simulink model "AUAV_V3_TestSensors_"  (R2015a)
settings: Solver=FixedStepDiscrete  StartTime=0.0  StopTime=10.0  FixedStep=T  RelTol=1e-3
PreLoadFcn:
  | %T = 0.0025;
  | MavlinkBus;
  | mcuInit;
  | % Baro Altitude Computation
  | % =========================
  | basePressure = 98192.64;
  | baseTemp = 288.215;
  | lapseRate = -0.00198122;
  | baseHeight = 0;
values from neighbouring files (symbols this model uses):
  apSampleTime = 0.01    [mcuInit.m]
  latlong_WP = 1    [mcuInit.m]
  mavlink_attitude_t = Simulink.Bus    [MavlinkBusMarcello.m]
  mavlink_gps_raw_int_t = Simulink.Bus    [MavlinkBus.m]    (also in MavlinkBusMarcello.m)
  mavlink_raw_imu_t = Simulink.Bus    [MavlinkBus.m]    (also in MavlinkBusMarcello.m)
  mavlink_scaled_pressure_t = Simulink.Bus    [MavlinkBus.m]    (also in MavlinkBusMarcello.m)
  mavlink_servo_output_raw_t = Simulink.Bus    [MavlinkBusMarcello.m]
  mavlink_sys_status_t = Simulink.Bus    [MavlinkBus.m]    (also in MavlinkBusMarcello.m)
  T = 0.01    [mcuInit.m]
  Xpoints = [0 0]    [mcuInit.m]
  Ypoints = [0 0]    [mcuInit.m]
  Zpoints = [0 0]    [mcuInit.m]
undefined symbols (not defined in the file or in its folder): A0, A14, A15, A2, A3, A4, A5, A6, accBiasRateLimit, B0, bankCommandLimit, barAdjust, baroCutoff, baroCutTemp, cubeAccelGain16405, cubeGyroGain16405, cubeMagGain16405, D0, D11, D7, D8, daLimit, data, daTrimMax, daTrimMin, deLimit, deTrimMax, deTrimMin, drLimit, drTrimMax, drTrimMin, dtLimit, dtTrimMax, dtTrimMin, F2, F3, G0, G13, G15, gaind, GS_location, gyroBiasRateLimit, IC1max, IPStar, ISA_g, Max, maxAcc, MaxDwnPthStar, maxDynPressure, maxEta, mlParamInterface, ms, OC1max, P112, P125, P127, P16, P20, P21, P30 ... (+26)
undefined symbols (not defined in the file): baroOffset, baroScale, barTGain1, barTGain2, barTMean1, barTMean2, bda, bde, bdr, bdt, bICda, bICde, bICdr, bICdt, derivativesConstant, lowRateSensorCutoff, mainSensorCutoff, mda, mde, mdr, mdt, mICda, mICde, mICdr, mICdt, pitotOffset, pitotScale, pitTGain1, pitTGain2, pitTMean1, pitTMean2, powerOffset, powerScale, pressureSensorCutoff, tempOffset, tempScale, vzCutoff, xCutoff, yCutoff
libraries: MCHP_Blockset x150, simulink x84, SLUGS_Library x31, aerolibconvert2 x6, aerolibutil x4, aerolibtransform2 x3, dspmtrx3 x2, aerolibobsolete x2
(part 11 of 20)

== system AUAV_V3_TestSensors_/Barometer_Driver/Baro Altimeter/Zero Out Height ==
  Base Height : Inport
  Computed Height : Inport  Port=2
  Enable : EnablePort
  Integer Delay : Delay  DelayLength=1  InitialCondition=0  InputProcessing=Inherited  SampleTime=.01
  Sum : Sum  Inputs=|+-  OutDataTypeStr=single
  Height Offset : Outport
  wires:
  Base Height/1 -> Sum/1
  Integer Delay/1 -> Sum/2
  Sum/1 -> Height Offset/1
  Computed Height/1 -> Integer Delay/1

== system AUAV_V3_TestSensors_/Barometer_Driver/I2C Initialisation Read EEPROM Calibration data Once (Blocking Function)/Pack10 ==
  Hi : Inport
  Low : Inport  Port=2
  Bitwise Operator : simulink/Logic and Bit Operations/Bitwise Operator  logicop=OR  UseBitMask=off  NumInputPorts=2  BitMask=bin2dec('11011001')  BitMaskRealWorld=Stored Integer
  Data Type Conversion1 : DataTypeConversion  OutDataTypeStr=uint16  ConvertRealWorld=Stored Integer (SI)
  Data Type Conversion2 : DataTypeConversion  OutDataTypeStr=uint16  ConvertRealWorld=Stored Integer (SI)
  Data Type Conversion3 : DataTypeConversion  OutDataTypeStr=uint16  ConvertRealWorld=Stored Integer (SI)
  Gain : Gain  Gain=2^8  OutDataTypeStr=Inherit: Same as input
  Out1 : Outport
  wires:
  Data Type Conversion3/1 -> Bitwise Operator/2
  Low/1 -> Data Type Conversion3/1
  Data Type Conversion1/1 -> Gain/1
  Bitwise Operator/1 -> Data Type Conversion2/1
  Hi/1 -> Data Type Conversion1/1
  Gain/1 -> Bitwise Operator/1
  Data Type Conversion2/1 -> Out1/1

== system AUAV_V3_TestSensors_/Barometer_Driver/I2C Initialisation Read EEPROM Calibration data Once (Blocking Function)/Pack11 ==
  Hi : Inport
  Low : Inport  Port=2
  Bitwise Operator : simulink/Logic and Bit Operations/Bitwise Operator  logicop=OR  UseBitMask=off  NumInputPorts=2  BitMask=bin2dec('11011001')  BitMaskRealWorld=Stored Integer
  Data Type Conversion1 : DataTypeConversion  OutDataTypeStr=uint16  ConvertRealWorld=Stored Integer (SI)
  Data Type Conversion2 : DataTypeConversion  OutDataTypeStr=uint16  ConvertRealWorld=Stored Integer (SI)
  Data Type Conversion3 : DataTypeConversion  OutDataTypeStr=uint16  ConvertRealWorld=Stored Integer (SI)
  Gain : Gain  Gain=2^8  OutDataTypeStr=Inherit: Same as input
  Out1 : Outport
  wires:
  Data Type Conversion3/1 -> Bitwise Operator/2
  Low/1 -> Data Type Conversion3/1
  Data Type Conversion1/1 -> Gain/1
  Bitwise Operator/1 -> Data Type Conversion2/1
  Hi/1 -> Data Type Conversion1/1
  Gain/1 -> Bitwise Operator/1
  Data Type Conversion2/1 -> Out1/1

== system AUAV_V3_TestSensors_/Barometer_Driver/I2C Initialisation Read EEPROM Calibration data Once (Blocking Function)/Pack12 ==
  Hi : Inport
  Low : Inport  Port=2
  Bitwise Operator : simulink/Logic and Bit Operations/Bitwise Operator  logicop=OR  UseBitMask=off  NumInputPorts=2  BitMask=bin2dec('11011001')  BitMaskRealWorld=Stored Integer
  Data Type Conversion1 : DataTypeConversion  OutDataTypeStr=uint16  ConvertRealWorld=Stored Integer (SI)
  Data Type Conversion2 : DataTypeConversion  OutDataTypeStr=uint16  ConvertRealWorld=Stored Integer (SI)
  Data Type Conversion3 : DataTypeConversion  OutDataTypeStr=uint16  ConvertRealWorld=Stored Integer (SI)
  Gain : Gain  Gain=2^8  OutDataTypeStr=Inherit: Same as input
  Out1 : Outport
  wires:
  Data Type Conversion2/1 -> Out1/1
  Gain/1 -> Bitwise Operator/1
  Hi/1 -> Data Type Conversion1/1
  Bitwise Operator/1 -> Data Type Conversion2/1
  Data Type Conversion1/1 -> Gain/1
  Low/1 -> Data Type Conversion3/1
  Data Type Conversion3/1 -> Bitwise Operator/2

== system AUAV_V3_TestSensors_/Barometer_Driver/I2C Initialisation Read EEPROM Calibration data Once (Blocking Function)/Pack2 ==
  Hi : Inport
  Low : Inport  Port=2
  Bitwise Operator : simulink/Logic and Bit Operations/Bitwise Operator  logicop=OR  UseBitMask=off  NumInputPorts=2  BitMask=bin2dec('11011001')  BitMaskRealWorld=Stored Integer
  Data Type Conversion1 : DataTypeConversion  OutDataTypeStr=uint16  ConvertRealWorld=Stored Integer (SI)
  Data Type Conversion2 : DataTypeConversion  OutDataTypeStr=uint16  ConvertRealWorld=Stored Integer (SI)
  Data Type Conversion3 : DataTypeConversion  OutDataTypeStr=uint16  ConvertRealWorld=Stored Integer (SI)
  Gain : Gain  Gain=2^8  OutDataTypeStr=Inherit: Same as input
  Out1 : Outport
  wires:
  Data Type Conversion2/1 -> Out1/1
  Gain/1 -> Bitwise Operator/1
  Hi/1 -> Data Type Conversion1/1
  Bitwise Operator/1 -> Data Type Conversion2/1
  Data Type Conversion1/1 -> Gain/1
  Low/1 -> Data Type Conversion3/1
  Data Type Conversion3/1 -> Bitwise Operator/2

== system AUAV_V3_TestSensors_/Barometer_Driver/I2C Initialisation Read EEPROM Calibration data Once (Blocking Function)/Pack3 ==
  Hi : Inport
  Low : Inport  Port=2
  Bitwise Operator : simulink/Logic and Bit Operations/Bitwise Operator  logicop=OR  UseBitMask=off  NumInputPorts=2  BitMask=bin2dec('11011001')  BitMaskRealWorld=Stored Integer
  Data Type Conversion1 : DataTypeConversion  OutDataTypeStr=uint16  ConvertRealWorld=Stored Integer (SI)
  Data Type Conversion2 : DataTypeConversion  OutDataTypeStr=uint16  ConvertRealWorld=Stored Integer (SI)
  Data Type Conversion3 : DataTypeConversion  OutDataTypeStr=uint16  ConvertRealWorld=Stored Integer (SI)
  Gain : Gain  Gain=2^8  OutDataTypeStr=Inherit: Same as input
  Out1 : Outport
  wires:
  Data Type Conversion3/1 -> Bitwise Operator/2
  Low/1 -> Data Type Conversion3/1
  Data Type Conversion1/1 -> Gain/1
  Bitwise Operator/1 -> Data Type Conversion2/1
  Hi/1 -> Data Type Conversion1/1
  Gain/1 -> Bitwise Operator/1
  Data Type Conversion2/1 -> Out1/1

== system AUAV_V3_TestSensors_/Barometer_Driver/I2C Initialisation Read EEPROM Calibration data Once (Blocking Function)/Pack4 ==
  Hi : Inport
  Low : Inport  Port=2
  Bitwise Operator : simulink/Logic and Bit Operations/Bitwise Operator  logicop=OR  UseBitMask=off  NumInputPorts=2  BitMask=bin2dec('11011001')  BitMaskRealWorld=Stored Integer
  Data Type Conversion1 : DataTypeConversion  OutDataTypeStr=uint16  ConvertRealWorld=Stored Integer (SI)
  Data Type Conversion2 : DataTypeConversion  OutDataTypeStr=uint16  ConvertRealWorld=Stored Integer (SI)
  Data Type Conversion3 : DataTypeConversion  OutDataTypeStr=uint16  ConvertRealWorld=Stored Integer (SI)
  Gain : Gain  Gain=2^8  OutDataTypeStr=Inherit: Same as input
  Out1 : Outport
  wires:
  Data Type Conversion3/1 -> Bitwise Operator/2
  Low/1 -> Data Type Conversion3/1
  Data Type Conversion1/1 -> Gain/1
  Bitwise Operator/1 -> Data Type Conversion2/1
  Hi/1 -> Data Type Conversion1/1
  Gain/1 -> Bitwise Operator/1
  Data Type Conversion2/1 -> Out1/1

== system AUAV_V3_TestSensors_/Barometer_Driver/I2C Initialisation Read EEPROM Calibration data Once (Blocking Function)/Pack5 ==
  Hi : Inport
  Low : Inport  Port=2
  Bitwise Operator : simulink/Logic and Bit Operations/Bitwise Operator  logicop=OR  UseBitMask=off  NumInputPorts=2  BitMask=bin2dec('11011001')  BitMaskRealWorld=Stored Integer
  Data Type Conversion1 : DataTypeConversion  OutDataTypeStr=uint16  ConvertRealWorld=Stored Integer (SI)
  Data Type Conversion2 : DataTypeConversion  OutDataTypeStr=uint16  ConvertRealWorld=Stored Integer (SI)
  Data Type Conversion3 : DataTypeConversion  OutDataTypeStr=uint16  ConvertRealWorld=Stored Integer (SI)
  Gain : Gain  Gain=2^8  OutDataTypeStr=Inherit: Same as input
  Out1 : Outport
  wires:
  Data Type Conversion2/1 -> Out1/1
  Gain/1 -> Bitwise Operator/1
  Hi/1 -> Data Type Conversion1/1
  Bitwise Operator/1 -> Data Type Conversion2/1
  Data Type Conversion1/1 -> Gain/1
  Low/1 -> Data Type Conversion3/1
  Data Type Conversion3/1 -> Bitwise Operator/2

== system AUAV_V3_TestSensors_/Barometer_Driver/I2C Initialisation Read EEPROM Calibration data Once (Blocking Function)/Pack6 ==
  Hi : Inport
  Low : Inport  Port=2
  Bitwise Operator : simulink/Logic and Bit Operations/Bitwise Operator  logicop=OR  UseBitMask=off  NumInputPorts=2  BitMask=bin2dec('11011001')  BitMaskRealWorld=Stored Integer
  Data Type Conversion1 : DataTypeConversion  OutDataTypeStr=uint16  ConvertRealWorld=Stored Integer (SI)
  Data Type Conversion2 : DataTypeConversion  OutDataTypeStr=uint16  ConvertRealWorld=Stored Integer (SI)
  Data Type Conversion3 : DataTypeConversion  OutDataTypeStr=uint16  ConvertRealWorld=Stored Integer (SI)
  Gain : Gain  Gain=2^8  OutDataTypeStr=Inherit: Same as input
  Out1 : Outport
  wires:
  Data Type Conversion3/1 -> Bitwise Operator/2
  Low/1 -> Data Type Conversion3/1
  Data Type Conversion1/1 -> Gain/1
  Bitwise Operator/1 -> Data Type Conversion2/1
  Hi/1 -> Data Type Conversion1/1
  Gain/1 -> Bitwise Operator/1
  Data Type Conversion2/1 -> Out1/1

== system AUAV_V3_TestSensors_/Barometer_Driver/I2C Initialisation Read EEPROM Calibration data Once (Blocking Function)/Pack7 ==
  Hi : Inport
  Low : Inport  Port=2
  Bitwise Operator : simulink/Logic and Bit Operations/Bitwise Operator  logicop=OR  UseBitMask=off  NumInputPorts=2  BitMask=bin2dec('11011001')  BitMaskRealWorld=Stored Integer
  Data Type Conversion1 : DataTypeConversion  OutDataTypeStr=uint16  ConvertRealWorld=Stored Integer (SI)
  Data Type Conversion2 : DataTypeConversion  OutDataTypeStr=uint16  ConvertRealWorld=Stored Integer (SI)
  Data Type Conversion3 : DataTypeConversion  OutDataTypeStr=uint16  ConvertRealWorld=Stored Integer (SI)
  Gain : Gain  Gain=2^8  OutDataTypeStr=Inherit: Same as input
  Out1 : Outport
  wires:
  Data Type Conversion2/1 -> Out1/1
  Gain/1 -> Bitwise Operator/1
  Hi/1 -> Data Type Conversion1/1
  Bitwise Operator/1 -> Data Type Conversion2/1
  Data Type Conversion1/1 -> Gain/1
  Low/1 -> Data Type Conversion3/1
  Data Type Conversion3/1 -> Bitwise Operator/2

== system AUAV_V3_TestSensors_/Barometer_Driver/I2C Initialisation Read EEPROM Calibration data Once (Blocking Function)/Pack8 ==
  Hi : Inport
  Low : Inport  Port=2
  Bitwise Operator : simulink/Logic and Bit Operations/Bitwise Operator  logicop=OR  UseBitMask=off  NumInputPorts=2  BitMask=bin2dec('11011001')  BitMaskRealWorld=Stored Integer
  Data Type Conversion1 : DataTypeConversion  OutDataTypeStr=uint16  ConvertRealWorld=Stored Integer (SI)
  Data Type Conversion2 : DataTypeConversion  OutDataTypeStr=uint16  ConvertRealWorld=Stored Integer (SI)
  Data Type Conversion3 : DataTypeConversion  OutDataTypeStr=uint16  ConvertRealWorld=Stored Integer (SI)
  Gain : Gain  Gain=2^8  OutDataTypeStr=Inherit: Same as input
  Out1 : Outport
  wires:
  Data Type Conversion2/1 -> Out1/1
  Gain/1 -> Bitwise Operator/1
  Hi/1 -> Data Type Conversion1/1
  Bitwise Operator/1 -> Data Type Conversion2/1
  Data Type Conversion1/1 -> Gain/1
  Low/1 -> Data Type Conversion3/1
  Data Type Conversion3/1 -> Bitwise Operator/2

== system AUAV_V3_TestSensors_/Barometer_Driver/I2C Initialisation Read EEPROM Calibration data Once (Blocking Function)/Pack9 ==
  Hi : Inport
  Low : Inport  Port=2
  Bitwise Operator : simulink/Logic and Bit Operations/Bitwise Operator  logicop=OR  UseBitMask=off  NumInputPorts=2  BitMask=bin2dec('11011001')  BitMaskRealWorld=Stored Integer
  Data Type Conversion1 : DataTypeConversion  OutDataTypeStr=uint16  ConvertRealWorld=Stored Integer (SI)
  Data Type Conversion2 : DataTypeConversion  OutDataTypeStr=uint16  ConvertRealWorld=Stored Integer (SI)
  Data Type Conversion3 : DataTypeConversion  OutDataTypeStr=uint16  ConvertRealWorld=Stored Integer (SI)
  Gain : Gain  Gain=2^8  OutDataTypeStr=Inherit: Same as input
  Out1 : Outport
  wires:
  Data Type Conversion3/1 -> Bitwise Operator/2
  Low/1 -> Data Type Conversion3/1
  Data Type Conversion1/1 -> Gain/1
  Bitwise Operator/1 -> Data Type Conversion2/1
  Hi/1 -> Data Type Conversion1/1
  Gain/1 -> Bitwise Operator/1
  Data Type Conversion2/1 -> Out1/1

== system AUAV_V3_TestSensors_/Control Surface Input/PilotConsole/Convert to Microseconds  ==
  IC : Inport
  Convert to Microseconds : Gain  Gain=0.2
  Data Type Conversion : DataTypeConversion  OutDataTypeStr=uint16
  uS : Outport
  wires:
  Convert to Microseconds/1 -> Data Type Conversion/1
  IC/1 -> Convert to Microseconds/1
  Data Type Conversion/1 -> uS/1

== system AUAV_V3_TestSensors_/Inner Loop// Navigation/Compute psi_dot_m/Protect NaNs ==
  In1 : Inport
  Integer Delay3 : Delay  DelayLength=1  InputProcessing=Inherited  SampleTime=T
  Relational Operator2 : RelationalOperator  Operator===  OutDataTypeStr=uint(8)
  Switch3 : Switch  Criteria=u2 > Threshold  Threshold=0.3  SampleTime=.01
  Out1 : Outport
  wires:
  Integer Delay3/1 -> Switch3/3
  Switch3/1 -> Out1/1, Integer Delay3/1
  In1/1 -> Relational Operator2/2, Relational Operator2/1, Switch3/1
  Relational Operator2/1 -> Switch3/2

== system AUAV_V3_TestSensors_/Inner Loop// Navigation/Compute psi_dot_m/dsPIC_cos ==
  u : Inport
  Environment Controller1 : simulink/Signal Routing/Environment Controller
  Trigonometric Function : Trigonometry  Operator=cos
  myCos() aLib.c [updated 5.1.16] : MCHP_Blockset/User Functions/C Function Call  ParseFilesChkbx=off  ListFunctions1=Custom Function  Function1=float myCos(float x)  AddHeaderDeclaration=off  Function1Type=when block is updated (default)  Fct1BlockIn=x  FctReturnBlockOut=on  DataCollected=0  ORDERING=None  SampleTime=-1  MCHP_MASTERLINK=|  PinDigitalInput=[]  PinDigitalOutput=[]  PinAnalogInput=[]
      | AUAV_V3_TestSensors_/Microchip Master
      | AUAV V3 Board
      | Busy Flag on D2 (RA6)
  cos(u) : Outport
  wires:
  u/1 -> Trigonometric Function/1, myCos() aLib.c [updated 5.1.16]/1
  Environment Controller1/1 -> cos(u)/1
  Trigonometric Function/1 -> Environment Controller1/1
  myCos() aLib.c [updated 5.1.16]/1 -> Environment Controller1/2

== system AUAV_V3_TestSensors_/Inner Loop// Navigation/Compute psi_dot_m/dsPIC_sin ==
  note: mySin()
      | alib.c
      | [updated 5.1.16]
  x : Inport
  C Function Call1 : MCHP_Blockset/User Functions/C Function Call  ParseFilesChkbx=off  ListFunctions1=Custom Function  Function1=float mySin(float x)  AddHeaderDeclaration=off  Function1Type=when block is updated (default)  Fct1BlockIn=x  FctReturnBlockOut=on  DataCollected=0  ORDERING=None  SampleTime=-1  MCHP_MASTERLINK=|  PinDigitalInput=[]  PinDigitalOutput=[]  PinAnalogInput=[]
      | AUAV_V3_TestSensors_/Microchip Master
      | AUAV V3 Board
      | Busy Flag on D2 (RA6)
  Environment Controller : simulink/Signal Routing/Environment Controller
  Trigonometric Function : Trigonometry
  sin(x) : Outport
  wires:
  x/1 -> Trigonometric Function/1, C Function Call1/1
  Trigonometric Function/1 -> Environment Controller/1
  Environment Controller/1 -> sin(x)/1
  C Function Call1/1 -> Environment Controller/2

== system AUAV_V3_TestSensors_/Inner Loop// Navigation/L1 Output Feedback Controller With Projection Operator/Control Law ==
  a : Inport
  u : Inport  Port=2
  Compute Coef : Subsystem
  Detect Change : Subsystem
  Divide : Product  SampleTime=apSampleTime
  Divide1 : Product  SampleTime=apSampleTime
  IC : InitialCondition
  Integer Delay : Delay  DelayLength=1  InputProcessing=Inherited  SampleTime=apSampleTime
  Integer Delay1 : Delay  DelayLength=1  InputProcessing=Inherited  SampleTime=apSampleTime
  Subtract : Sum  SampleTime=apSampleTime
  y : Outport
  wires:
  a/1 -> Compute Coef/1(a), Detect Change/1(Data)
  Compute Coef/1(b) -> Divide/1
  Compute Coef/2(c) -> Divide1/1
  Detect Change/1(change?) -> IC/1
  Integer Delay/1 -> Divide/2
  Divide/1 -> Subtract/1
  Divide1/1 -> Subtract/2
  Subtract/1 -> y/1, Integer Delay1/1
  IC/1 -> Compute Coef/Enable
  u/1 -> Integer Delay/1
  Integer Delay1/1 -> Divide1/2

== system AUAV_V3_TestSensors_/Inner Loop// Navigation/L1 Output Feedback Controller With Projection Operator/Projection Operator ==
  Theta Max : Inport
  Eps 0 : Inport  Port=2
  Theta : Inport  Port=3
  y : Inport  Port=4
  Compare To Zero : simulink/Logic and Bit Operations/Compare To Zero  relop=>=  OutDataTypeStr=boolean  ZeroCross=off
  Compare To Zero1 : simulink/Logic and Bit Operations/Compare To Zero  relop=>  OutDataTypeStr=boolean  ZeroCross=off
  Divide2 : Product  OutDataTypeStr=single
  Enabled Subsystem : Subsystem  TreatAsAtomicUnit=on
  Enabled Subsystem1 : Subsystem  TreatAsAtomicUnit=on
  F(theta) : Subsystem
  Logical Operator : Logic  Operator=NOT  AllPortsSameDT=off  OutDataTypeStr=uint(8)
  Logical Operator2 : Logic  AllPortsSameDT=off  OutDataTypeStr=uint(8)
  Merge : Merge  InitialOutput=0
  "y " : InportShadow  Port=4
  "y    " : InportShadow  Port=4
  "Proj(the, y)" : Outport
  wires:
  Theta Max/1 -> F(theta)/1(Theta Max)
  Eps 0/1 -> F(theta)/2(Eps 0)
  Theta/1 -> F(theta)/3(Theta)
  F(theta)/1(f_theta) -> Compare To Zero/1, Enabled Subsystem1/2(f_the)
  y/1 -> Divide2/2
  Divide2/1 -> Compare To Zero1/1
  Merge/1 -> "Proj(the, y)"/1
  "y "/1 -> Enabled Subsystem/1(In1)
  Enabled Subsystem/1(Out1) -> Merge/1
  Compare To Zero/1 -> Logical Operator2/2
  F(theta)/2(dif_f_theta) -> Divide2/1, Enabled Subsystem1/3(grad)
  Compare To Zero1/1 -> Logical Operator2/1
  Logical Operator2/1 -> Logical Operator/1, Enabled Subsystem1/Enable
  Logical Operator/1 -> Enabled Subsystem/Enable
  "y    "/1 -> Enabled Subsystem1/1(y)
  Enabled Subsystem1/1(Out1) -> Merge/2

== system AUAV_V3_TestSensors_/Inner Loop// Navigation/L1 Output Feedback Controller With Projection Operator/Protect NaNs ==
  In1 : Inport
  Integer Delay3 : Delay  DelayLength=1  InputProcessing=Inherited  SampleTime=T
  Relational Operator2 : RelationalOperator  Operator===  OutDataTypeStr=uint(8)
  Switch3 : Switch  Criteria=u2 > Threshold  Threshold=0.3  SampleTime=.01
  Out1 : Outport
  wires:
  Relational Operator2/1 -> Switch3/2
  In1/1 -> Switch3/1, Relational Operator2/1, Relational Operator2/2
  Switch3/1 -> Integer Delay3/1, Out1/1
  Integer Delay3/1 -> Switch3/3

== system AUAV_V3_TestSensors_/Inner Loop// Navigation/L1 Output Feedback Controller With Projection Operator/Protect NaNs2 ==
  In1 : Inport
  Integer Delay3 : Delay  DelayLength=1  InputProcessing=Inherited  SampleTime=T
  Relational Operator2 : RelationalOperator  Operator===  OutDataTypeStr=uint(8)
  Switch3 : Switch  Criteria=u2 > Threshold  Threshold=0.3  SampleTime=.01
  Out1 : Outport
  wires:
  Relational Operator2/1 -> Switch3/2
  In1/1 -> Switch3/1, Relational Operator2/1, Relational Operator2/2
  Switch3/1 -> Integer Delay3/1, Out1/1
  Integer Delay3/1 -> Switch3/3

== system AUAV_V3_TestSensors_/Inner Loop// Navigation/L1 Output Feedback Controller With Projection Operator/State Predictor ==
  a : Inport
  u : Inport  Port=2
  Compute Coef : Subsystem
  Detect Change : Subsystem
  Divide : Product  SampleTime=apSampleTime
  Divide1 : Product  SampleTime=apSampleTime
  IC : InitialCondition
  Integer Delay : Delay  DelayLength=1  InputProcessing=Inherited  SampleTime=apSampleTime
  Integer Delay1 : Delay  DelayLength=1  InputProcessing=Inherited  SampleTime=apSampleTime
  Subtract : Sum  SampleTime=apSampleTime
  y : Outport
  wires:
  Integer Delay1/1 -> Divide1/2
  u/1 -> Integer Delay/1
  IC/1 -> Compute Coef/Enable
  Subtract/1 -> Integer Delay1/1, y/1
  Divide1/1 -> Subtract/2
  Divide/1 -> Subtract/1
  Integer Delay/1 -> Divide/2
  Detect Change/1(change?) -> IC/1
  Compute Coef/2(c) -> Divide1/1
  Compute Coef/1(b) -> Divide/1
  a/1 -> Detect Change/1(Data), Compute Coef/1(a)

== system AUAV_V3_TestSensors_/Inner Loop// Navigation/L1 Output Feedback Controller With Projection Operator/Trapezoidal Integrator ==
  x : Inport
  Reset : Inport  Port=2
  Constant : Constant  Value=1/3  OutDataTypeStr=single
  Constant1 : Constant  Value=4/3  OutDataTypeStr=single
  Constant2 : Constant  Value=T/2  OutDataTypeStr=single
  Constant3 : Constant  Value=1/3  OutDataTypeStr=single
  Constant5 : Constant  Value=0  OutDataTypeStr=single
  Integer Delay : Delay  DelayLength=1  InputProcessing=Inherited  SampleTime=T
  Integer Delay1 : Delay  InputProcessing=Inherited  SampleTime=T
  Integer Delay2 : Delay  DelayLength=1  InputProcessing=Inherited  SampleTime=T
  Product{,1..3} (4 alike) : Product  OutDataTypeStr=single  RndMeth=Zero
  Protect NaNs : Subsystem
  Protect NaNs1 : Subsystem
  Subtract : Sum  Inputs=3  OutDataTypeStr=single
  Subtract1 : Sum  Inputs=2  OutDataTypeStr=single
  Switch1 : Switch  Criteria=u2 > Threshold  Threshold=0.3  SampleTime=.01
  "[min max]" : Saturate  UpperLimit=upperLimit  LowerLimit=lowerLimit  SampleTime=T
  Int(x) : Outport
  wires:
  Constant/1 -> Product/2
  Constant1/1 -> Product1/2
  Integer Delay/1 -> Product1/1
  Integer Delay1/1 -> Product2/1
  Constant3/1 -> Product2/2
  x/1 -> Protect NaNs/1(In1)
  Product/1 -> Subtract/1
  Product1/1 -> Subtract/2
  Product2/1 -> Subtract/3
  Constant2/1 -> Product3/1
  Subtract/1 -> Product3/2
  Integer Delay2/1 -> Subtract1/1
  Constant5/1 -> Switch1/1
  Reset/1 -> Switch1/2
  Switch1/1 -> Protect NaNs1/1(In1)
  "[min max]"/1 -> Switch1/3
  Product3/1 -> Subtract1/2
  Subtract1/1 -> "[min max]"/1
  Protect NaNs/1(Out1) -> Product/1, Integer Delay/1, Integer Delay1/1
  Protect NaNs1/1(Out1) -> Int(x)/1, Integer Delay2/1

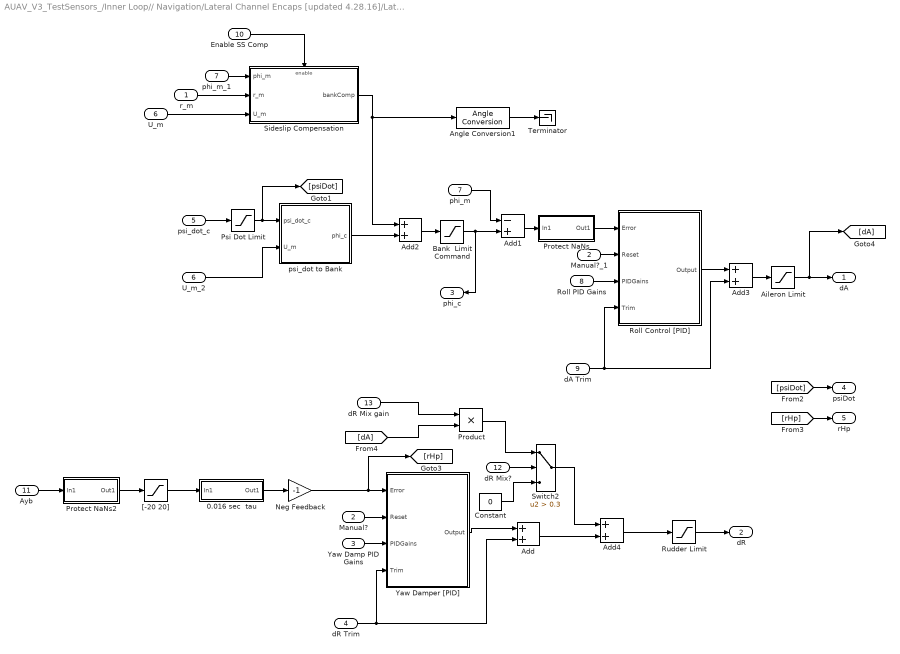
== system AUAV_V3_TestSensors_/Inner Loop// Navigation/Lateral Channel Encaps [updated 4.28.16]/Lateral Channel ==
  r_m : Inport
  Manual? : Inport  Port=2
  Yaw Damp PID Gains : Inport  Port=3
  dR Trim : Inport  Port=4
  psi_dot_c : Inport  Port=5
  U_m : Inport  Port=6
  phi_m : Inport  Port=7
  Roll PID Gains : Inport  Port=8
  dA Trim : Inport  Port=9
  Enable SS Comp : Inport  Port=10
  Ayb : Inport  Port=11
  dR Mix? : Inport  Port=12
  dR Mix gain : Inport  Port=13
  0.016 sec  tau : Subsystem  mask(Tustin1stOrderLowpassAutoInitialCondition){f=10, T=T}
      mask prompts: f "Lowpass Frequency"; T "Sample Time"
      mask help: Takes a 3db rolloff frequency (in Hz, NOT radians/s) and a sample time. Performs a symbolic Tustin conversion and implements in a discrete filter. The initial output of the filter is set by the first sample.
      mask Help: Enter the desired 3db rolloff frequency in Hz and the sample time. Initial conditions are sampled automatically.
      mask Display: fprintf('%.2f Hz lowpass',f)
  Add{,2..4} (4 alike) : Sum  OutDataTypeStr=single
  Add1 : Sum  Inputs=-+  OutDataTypeStr=single
  Aileron Limit : Saturate  UpperLimit=daLimit  LowerLimit=-daLimit  SampleTime=apSampleTime
  Angle Conversion1 : aerolibconvert2/Angle Conversion  IU=rad  OU=deg
  Bank  Limit Command : Saturate  UpperLimit=bankCommandLimit  LowerLimit=-bankCommandLimit  SampleTime=apSampleTime
  Constant : Constant  Value=0  OutDataTypeStr=single
  Manual?_1 : InportShadow  Port=2
  "Neg Feedback " : Gain  Gain=-1  OutDataTypeStr=float('single')
  Product : Product  RndMeth=Zero
  Protect NaNs : Subsystem
  Protect NaNs2 : Subsystem
  Psi Dot Limit : Saturate  UpperLimit=1  LowerLimit=-1  SampleTime=apSampleTime
  Roll Control [PID] : Subsystem  AncestorBlock=SLUGS_Library/Control Blocks/PID Controller w//Anti-Windup  mask(PID){Tsample=apSampleTime, Ndelay=derivativesConstant, upperSaturationLimit=daLimit, lowerSaturationLimit=-daLimit}
      mask prompts: Tsample "Sample Time"; Ndelay "Integer delays for de/dt"; upperSaturationLimit "Upper Saturation Limit"; lowerSaturationLimit "Lower Saturation Limit"
      mask help: PID controller block with anti-windup and saturation limits. Implemented as a discrete forwardl integration which stops integrating when the output is saturated. Derivative is implemented as a numerical derivative with N integer delays to smooth output.
      mask Display:
      | disp('PID')
      | port_label('input',1,'error')
      | port_label('input',3,'gains')
      | port_label('input',2,'reset')
      | port_label('input',4,'trim')
      | port_label('output',1,'output')
  Rudder Limit : Saturate  UpperLimit=drLimit  LowerLimit=-drLimit  SampleTime=apSampleTime
  Sideslip Compensation : Subsystem
  Switch2 : Switch  Criteria=u2 > Threshold  Threshold=0.3  InputSameDT=on
  Terminator : Terminator
  U_m_2 : InportShadow  Port=6
  Yaw Damper [PID] : Subsystem  AncestorBlock=SLUGS_Library/Control Blocks/PID Controller w//Anti-Windup  mask(PID){Tsample=apSampleTime, Ndelay=derivativesConstant, upperSaturationLimit=drLimit, lowerSaturationLimit=-drLimit}
      mask prompts: Tsample "Sample Time"; Ndelay "Integer delays for de/dt"; upperSaturationLimit "Upper Saturation Limit"; lowerSaturationLimit "Lower Saturation Limit"
      mask help: PID controller block with anti-windup and saturation limits. Implemented as a discrete forwardl integration which stops integrating when the output is saturated. Derivative is implemented as a numerical derivative with N integer delays to smooth output.
      mask Display:
      | disp('PID')
      | port_label('input',1,'error')
      | port_label('input',3,'gains')
      | port_label('input',2,'reset')
      | port_label('input',4,'trim')
      | port_label('output',1,'output')
  "[-20 20]" : Saturate  UpperLimit=20  LowerLimit=-20
  phi_m_1 : InportShadow  Port=7
  psi_dot to Bank : Subsystem  AncestorBlock=SLUGS_Library/Navigation/psi_dot to Bank
  dA : Outport
  dR : Outport  Port=2
  phi_c : Outport  Port=3
  psiDot : Outport  Port=4
  rHp : Outport  Port=5
  wires:
  [rHp] -> rHp/1
  [psiDot] -> psiDot/1
  [dA] -> Product/2
  dR Mix gain/1 -> Product/1
  Product/1 -> Switch2/1
  Constant/1 -> Switch2/3
  dR Mix?/1 -> Switch2/2
  Switch2/1 -> Add4/1
  Add/1 -> Add4/2
  Add4/1 -> Rudder Limit/1
  Angle Conversion1/1 -> Terminator/1
  "[-20 20]"/1 -> 0.016 sec  tau/1(In1)
  Protect NaNs2/1(Out1) -> "[-20 20]"/1
  Protect NaNs/1(Out1) -> Roll Control [PID]/1(Error)
  Rudder Limit/1 -> dR/1
  0.016 sec  tau/1(Out1) -> "Neg Feedback "/1
  "Neg Feedback "/1 -> Yaw Damper [PID]/1(Error), [rHp]
  Ayb/1 -> Protect NaNs2/1(In1)
  Enable SS Comp/1 -> Sideslip Compensation/Enable
  U_m/1 -> Sideslip Compensation/3(U_m)
  r_m/1 -> Sideslip Compensation/2(r_m)
  phi_m_1/1 -> Sideslip Compensation/1(phi_m)
  Sideslip Compensation/1(bankComp) -> Angle Conversion1/1, Add2/1
  psi_dot to Bank/1(phi_c) -> Add2/2
  Add2/1 -> Bank  Limit Command/1
  U_m_2/1 -> psi_dot to Bank/2(U_m)
  Manual?/1 -> Yaw Damper [PID]/2(Reset)
  Yaw Damp PID Gains/1 -> Yaw Damper [PID]/3(PIDGains)
  Yaw Damper [PID]/1(Output) -> Add/1
  dR Trim/1 -> Yaw Damper [PID]/4(Trim), Add/2
  Manual?_1/1 -> Roll Control [PID]/2(Reset)
  Roll PID Gains/1 -> Roll Control [PID]/3(PIDGains)
  Add3/1 -> Aileron Limit/1
  Roll Control [PID]/1(Output) -> Add3/1
  dA Trim/1 -> Roll Control [PID]/4(Trim), Add3/2
  Aileron Limit/1 -> [dA], dA/1
  Add1/1 -> Protect NaNs/1(In1)
  phi_m/1 -> Add1/1
  Bank  Limit Command/1 -> phi_c/1, Add1/2
  Psi Dot Limit/1 -> [psiDot], psi_dot to Bank/1(psi_dot_c)
  psi_dot_c/1 -> Psi Dot Limit/1

== system AUAV_V3_TestSensors_/Inner Loop// Navigation/Lateral Channel Encaps [updated 4.28.16]/psi_dot_c Select logic1 ==
  psi_dot_ad : Inport
  L1OnOff : Inport  Port=2
  psi_dot_c_noNav : Inport  Port=3
  IsPassThrough : Inport  Port=4
  nav_phi_c : Inport  Port=5
  U_m : Inport  Port=6
  Bank to Psi Dot : Subsystem  AncestorBlock=SLUGS_Library/Navigation/Bank to Psi Dot
  Switch : Switch  Criteria=u2 > Threshold  Threshold=0.3
  Switch1 : Switch  Criteria=u2 > Threshold  Threshold=0.3  InputSameDT=on
  psi_dot_c : Outport
  psi_dot_c_4_L1 : Outport  Port=2
  wires:
  U_m/1 -> Bank to Psi Dot/2(U_m)
  nav_phi_c/1 -> Bank to Psi Dot/1(phi_c)
  IsPassThrough/1 -> Switch1/2
  psi_dot_c_noNav/1 -> Switch1/1
  Switch/1 -> psi_dot_c/1
  L1OnOff/1 -> Switch/2
  psi_dot_ad/1 -> Switch/1
  Switch1/1 -> psi_dot_c_4_L1/1, Switch/3
  Bank to Psi Dot/1(psi_dot_c) -> Switch1/3

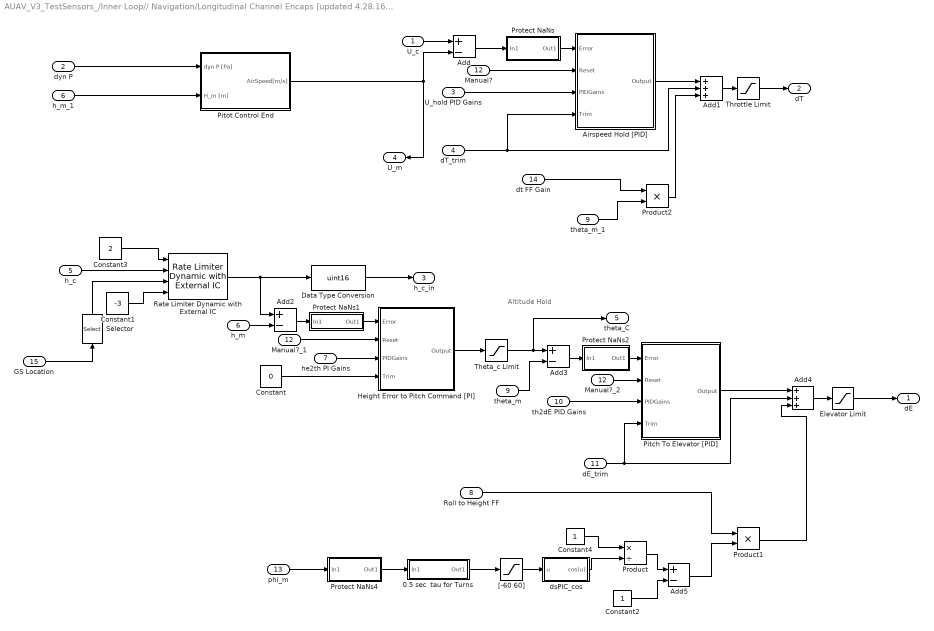
== system AUAV_V3_TestSensors_/Inner Loop// Navigation/Longitudinal Channel Encaps [updated 4.28.16]/Longitudinal Channel ==
  note: Altitude Hold
  U_c : Inport
  dyn P : Inport  Port=2
  U_hold PID Gains : Inport  Port=3
  dT_trim : Inport  Port=4
  h_c : Inport  Port=5
  h_m : Inport  Port=6
  he2th PI Gains : Inport  Port=7
  Roll to Height FF : Inport  Port=8
  theta_m : Inport  Port=9
  th2dE PID Gains : Inport  Port=10
  dE_trim : Inport  Port=11
  Manual? : Inport  Port=12
  phi_m : Inport  Port=13
  dt FF Gain : Inport  Port=14
  GS Location : Inport  Port=15
  0.5 sec  tau for Turns : Subsystem  mask(Tustin1stOrderLowpassAutoInitialCondition){f=0.32, T=T}
      mask prompts: f "Lowpass Frequency"; T "Sample Time"
      mask help: Takes a 3db rolloff frequency (in Hz, NOT radians/s) and a sample time. Performs a symbolic Tustin conversion and implements in a discrete filter. The initial output of the filter is set by the first sample.
      mask Help: Enter the desired 3db rolloff frequency in Hz and the sample time. Initial conditions are sampled automatically.
      mask Display: fprintf('%.2f Hz lowpass',f)
  Add : Sum  Inputs=+-
  Add1 : Sum  Inputs=3  OutDataTypeStr=single
  Add2 : Sum  Inputs=+-  OutDataTypeStr=single
  Add3 : Sum  Inputs=+-  OutDataTypeStr=single
  Add4 : Sum  Inputs=3  OutDataTypeStr=single
  Add5 : Sum  Inputs=+-  OutDataTypeStr=single
  Airspeed Hold [PID] : Subsystem  AncestorBlock=SLUGS_Library/Control Blocks/PID Controller w//Anti-Windup  mask(PID){Tsample=apSampleTime, Ndelay=derivativesConstant, upperSaturationLimit=dtLimit, lowerSaturationLimit=0}
      mask prompts: Tsample "Sample Time"; Ndelay "Integer delays for de/dt"; upperSaturationLimit "Upper Saturation Limit"; lowerSaturationLimit "Lower Saturation Limit"
      mask help: PID controller block with anti-windup and saturation limits. Implemented as a discrete forwardl integration which stops integrating when the output is saturated. Derivative is implemented as a numerical derivative with N integer delays to smooth output.
      mask Display:
      | disp('PID')
      | port_label('input',1,'error')
      | port_label('input',3,'gains')
      | port_label('input',2,'reset')
      | port_label('input',4,'trim')
      | port_label('output',1,'output')
  Constant : Constant  Value=0
  Constant1 : Constant  Value=-3  OutDataTypeStr=single
  Constant2 : Constant  OutDataTypeStr=single
  Constant3 : Constant  Value=2  OutDataTypeStr=single
  Constant4 : Constant  OutDataTypeStr=single
  Data Type Conversion : DataTypeConversion  OutDataTypeStr=uint16
  Elevator Limit : Saturate  UpperLimit=deLimit  LowerLimit=-deLimit  SampleTime=apSampleTime
  Height Error to Pitch Command [PI] : Subsystem  AncestorBlock=SLUGS_Library/Control Blocks/PI Controller w//Anti-Windup  mask(PID){Tsample=apSampleTime, Ndelay=derivativesConstant, upperSaturationLimit=pitchCommandLimit, lowerSaturationLimit=-pitchCommandLimit}
      mask prompts: Tsample "Sample Time"; Ndelay "Integer delays for de/dt"; upperSaturationLimit "Upper Saturation Limit"; lowerSaturationLimit "Lower Saturation Limit"
      mask help: PID controller block with anti-windup and saturation limits. Implemented as a discrete forwardl integration which stops integrating when the output is saturated. Derivative is implemented as a numerical derivative with N integer delays to smooth output.
      mask Display:
      | disp('PI')
      | port_label('input',1,'error')
      | port_label('input',3,'gains')
      | port_label('input',2,'reset')
      | port_label('input',4,'trim')
      | port_label('output',1,'output')
  Manual?_1 : InportShadow  Port=12
  Manual?_2 : InportShadow  Port=12
  Pitch To Elevator [PID] : Subsystem  AncestorBlock=SLUGS_Library/Control Blocks/PID Controller w//Anti-Windup  mask(PID){Tsample=apSampleTime, Ndelay=derivativesConstant, upperSaturationLimit=deLimit, lowerSaturationLimit=-deLimit}
      mask prompts: Tsample "Sample Time"; Ndelay "Integer delays for de/dt"; upperSaturationLimit "Upper Saturation Limit"; lowerSaturationLimit "Lower Saturation Limit"
      mask help: PID controller block with anti-windup and saturation limits. Implemented as a discrete forwardl integration which stops integrating when the output is saturated. Derivative is implemented as a numerical derivative with N integer delays to smooth output.
      mask Display:
      | disp('PID')
      | port_label('input',1,'error')
      | port_label('input',3,'gains')
      | port_label('input',2,'reset')
      | port_label('input',4,'trim')
      | port_label('output',1,'output')
  Pitot Control End : Subsystem  AncestorBlock=SLUGS_Library/Sensor Blocks/Pitot Control End
  Product : Product  Inputs=*/  RndMeth=Zero
  Product1 : Product  RndMeth=Zero
  Product2 : Product  RndMeth=Zero
  Protect NaNs : Subsystem
  Protect NaNs1 : Subsystem
  Protect NaNs2 : Subsystem
  Protect NaNs4 : Subsystem
  Rate Limiter Dynamic with External IC : SLUGS_Library/Singnal Routing & Conditioning/Rate Limiter Dynamic with External IC  rlIC=0
  Selector : Selector  InputPortWidth=3  Indices=[1 ]
  Theta_c Limit : Saturate  UpperLimit=pitchCommandLimit  LowerLimit=-pitchCommandLimit  SampleTime=apSampleTime
  Throttle Limit : Saturate  UpperLimit=dtLimit  LowerLimit=0  SampleTime=apSampleTime
  "[-60 60]" : Saturate  UpperLimit=60  LowerLimit=-60  SampleTime=apSampleTime
  dsPIC_cos : Subsystem  AncestorBlock=SLUGS_Library/dsPIC_cos
  h_m_1 : InportShadow  Port=6
  theta_m_1 : InportShadow  Port=9
  dE : Outport
  dT : Outport  Port=2
  h_c_in : Outport  Port=3
  U_m : Outport  Port=4
  theta_C : Outport  Port=5
  wires:
  GS Location/1 -> Selector/1
  Protect NaNs4/1(Out1) -> 0.5 sec  tau for Turns/1(In1)
  Protect NaNs2/1(Out1) -> Pitch To Elevator [PID]/1(Error)
  Protect NaNs1/1(Out1) -> Height Error to Pitch Command [PI]/1(Error)
  Protect NaNs/1(Out1) -> Airspeed Hold [PID]/1(Error)
  Constant/1 -> Height Error to Pitch Command [PI]/4(Trim)
  U_hold PID Gains/1 -> Airspeed Hold [PID]/3(PIDGains)
  dt FF Gain/1 -> Product2/1
  Product2/1 -> Add1/3
  theta_m_1/1 -> Product2/2
  Product1/1 -> Add4/3
  Roll to Height FF/1 -> Product1/1
  Add5/1 -> Product1/2
  "[-60 60]"/1 -> dsPIC_cos/1(u)
  0.5 sec  tau for Turns/1(Out1) -> "[-60 60]"/1
  Product/1 -> Add5/1
  Constant4/1 -> Product/1
  dsPIC_cos/1(cos(u)) -> Product/2
  Constant2/1 -> Add5/2
  phi_m/1 -> Protect NaNs4/1(In1)
  Pitot Control End/1(AirSpeed[m/s]) -> U_m/1, Add/2
  U_c/1 -> Add/1
  Add/1 -> Protect NaNs/1(In1)
  Airspeed Hold [PID]/1(Output) -> Add1/1
  dT_trim/1 -> Airspeed Hold [PID]/4(Trim), Add1/2
  Add1/1 -> Throttle Limit/1
  Throttle Limit/1 -> dT/1
  Add2/1 -> Protect NaNs1/1(In1)
  h_m/1 -> Add2/2
  theta_m/1 -> Add3/2
  Manual?/1 -> Airspeed Hold [PID]/2(Reset)
  Manual?_1/1 -> Height Error to Pitch Command [PI]/2(Reset)
  Manual?_2/1 -> Pitch To Elevator [PID]/2(Reset)
  Add4/1 -> Elevator Limit/1
  Pitch To Elevator [PID]/1(Output) -> Add4/1
  dE_trim/1 -> Pitch To Elevator [PID]/4(Trim), Add4/2
  Elevator Limit/1 -> dE/1
  dyn P/1 -> Pitot Control End/1(dyn P [Pa])
  h_m_1/1 -> Pitot Control End/2(H_m [m])
  he2th PI Gains/1 -> Height Error to Pitch Command [PI]/3(PIDGains)
  th2dE PID Gains/1 -> Pitch To Elevator [PID]/3(PIDGains)
  Add3/1 -> Protect NaNs2/1(In1)
  Theta_c Limit/1 -> theta_C/1, Add3/1
  Rate Limiter Dynamic with External IC/1 -> Data Type Conversion/1, Add2/1
  Height Error to Pitch Command [PI]/1(Output) -> Theta_c Limit/1
  Constant3/1 -> Rate Limiter Dynamic with External IC/1
  Selector/1 -> Rate Limiter Dynamic with External IC/3
  Constant1/1 -> Rate Limiter Dynamic with External IC/4
  h_c/1 -> Rate Limiter Dynamic with External IC/2
  Data Type Conversion/1 -> h_c_in/1
